simulink model "sim_discrete_planar_7dof"  (R2023b)
settings: Solver=VariableStepAuto  StartTime=0.0  StopTime=T_sim  FixedStep=param_global.Ta  RelTol=1e-3
InitFcn:
  | parameters_7dof;
undefined symbols (not defined in the file): fx, fy, fz, init_bus_param, param_global, param_robot, param_vis, path_param, q_0, q_0_p, tau_x, tau_y, tau_z
(part 1 of 2)
settings Model: Creator=emu  LastModifiedBy=emu
settings DebuggingCC: ReadBeforeWriteMsg=DisableAll  WriteAfterWriteMsg=DisableAll  WriteAfterReadMsg=DisableAll  MultiTaskDSMMsg=none
settings ModelReferenceCC: UpdateModelReferenceTargets=IfOutOfDate
settings SFSimCC: SFSimEcho=off

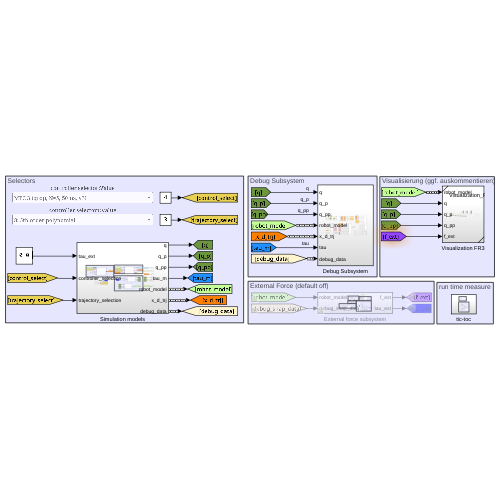
[thumbnail: Simulink's stored preview of the top-level diagram]
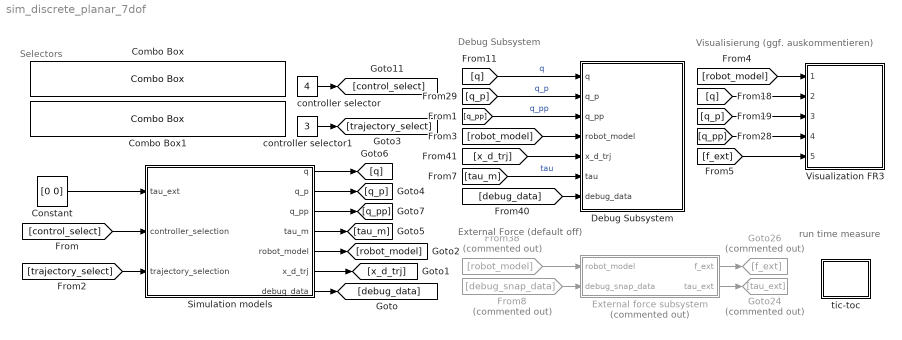
== system sim_discrete_planar_7dof ==
  note: run time measure
  note: Selectors
  note: Visualisierung (ggf. auskommentieren)
  note: Debug Subsystem
  note: External Force (default off)
  Combo Box : ComboBox  SelectedLabel=MPC 3 (qrqp, N=5, 50ms, v3)
      settings: Values={{'Cartesian CT Control', 'MPC 1 (ipopt, N=5, 20ms, v2)', 'MPC 2 (qrqp, N=5, 20ms, v2)', 'MPC 3 (qrqp, N=5, 50ms, v3)', 'MPC 4 (qrqp, N=5, 1ms, v1)', 'MPC 5 (qrqp, N=5, 10ms, v4'}, [1 2 3 4 5 6]}
  Combo Box1 : ComboBox  SelectedLabel=3: 5th order polynomial
      settings: Values={{'1: stabilize equilibrium', '2: 5th order differential filter', '3: 5th order polynomial', '4: smooth sinus'}, [1 2 3 4]}
  Constant : Constant  Value=[0 0]
  Debug Subsystem : Subsystem
  External force subsystem : Subsystem  Commented=on
  From38 : From  Commented=on  GotoTag=robot_model
  From8 : From  Commented=on  GotoTag=debug_snap_data
  Goto24 : Goto  Commented=on  GotoTag=tau_ext
  Goto26 : Goto  Commented=on  GotoTag=f_ext
  Simulation models : Subsystem
  Visualization FR3 : Subsystem  ReferencedSubsystem=Visualization_FR3_shared_subsystem
  controller selector : Constant  Value=4  OutDataTypeStr=uint32  SampleTime=-1
  controller selector1 : Constant  Value=3  OutDataTypeStr=uint32  SampleTime=-1
  tic-toc : Subsystem
  wires:
  controller selector/1 -> [control_select]
  [tau_m] -> Debug Subsystem/6(tau)  "tau"
  [debug_data] -> Debug Subsystem/7(debug_data)
  External force subsystem/1(f_ext) -> Goto26/1
  [q_p] -> Debug Subsystem/2(q_p)  "q_p"
  [robot_model] -> Debug Subsystem/4(robot_model)
  [robot_model] -> Visualization FR3/1
  From8/1 -> External force subsystem/2(debug_snap_data)
  [q_pp] -> Visualization FR3/4
  [f_ext] -> Visualization FR3/5
  [x_d_trj] -> Debug Subsystem/5(x_d_trj)
  From38/1 -> External force subsystem/1(robot_model)
  [q_p] -> Visualization FR3/3
  External force subsystem/2(tau_ext) -> Goto24/1
  [q] -> Visualization FR3/2
  [q] -> Debug Subsystem/1(q)  "q"
  [q_pp] -> Debug Subsystem/3(q_pp)  "q_pp"
  Simulation models/7(debug_data) -> [debug_data]
  Simulation models/6(x_d_trj) -> [x_d_trj]
  Simulation models/5(robot_model) -> [robot_model]
  Simulation models/4(tau_m) -> [tau_m]
  Simulation models/3(q_pp) -> [q_pp]
  Simulation models/2(q_p) -> [q_p]
  Simulation models/1(q) -> [q]
  [control_select] -> Simulation models/2(controller_selection)
  Constant/1 -> Simulation models/1(tau_ext)
  controller selector1/1 -> [trajectory_select]
  [trajectory_select] -> Simulation models/3(trajectory_selection)

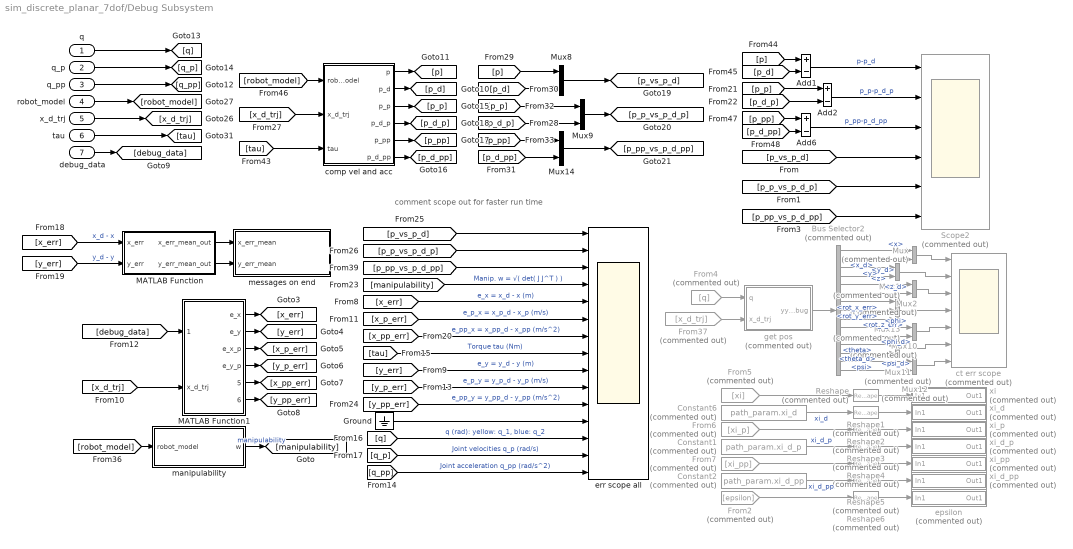
== system sim_discrete_planar_7dof/Debug Subsystem ==
  note: comment scope out for faster run time
  q : Inport
  q_p : Inport  Port=2
  q_pp : Inport  Port=3
  robot_model : Inport  Port=4
  x_d_trj : Inport  Port=5
  tau : Inport  Port=6
  debug_data : Inport  Port=7  OutDataTypeStr=Bus: debug_data_bus
  Add1 : Sum  Inputs=+-
  Add2 : Sum  Inputs=+-
  Add6 : Sum  Inputs=+-
  Bus Selector2 : BusSelector  Commented=on  OutputSignals=x,x_d,y,y_d,z,z_d,rot_x_err,rot_y_err,rot_z_err,phi,phi_d,theta,theta_d,psi,psi_d
  Constant1 : Constant  Commented=on  Value=path_param.xi_d_p  SampleTime=-1
  Constant2 : Constant  Commented=on  Value=path_param.xi_d_pp  SampleTime=-1
  Constant6 : Constant  Commented=on  Value=path_param.xi_d  SampleTime=-1
  From2 : From  Commented=on  GotoTag=epsilon
  From37 : From  Commented=on  GotoTag=x_d_trj
  From4 : From  Commented=on  GotoTag=q
  From5 : From  Commented=on  GotoTag=xi
  From6 : From  Commented=on  GotoTag=xi_p
  From7 : From  Commented=on  GotoTag=xi_pp
  Ground : Ground
  MATLAB Function : MATLAB Function  TreatAsAtomicUnit=on
  MATLAB Function1 : MATLAB Function  TreatAsAtomicUnit=on
  Mux{,1..2,10..12} (6 alike) : Mux  Commented=on  Inputs=2
  Mux13 : Mux  Commented=on  Inputs=3
  Mux14 : Mux  Inputs=2
  Mux8 : Mux  Inputs=2
  Mux9 : Mux  Inputs=2
  Reshape{,1..6} (7 alike) : Reshape  Commented=on
  Scope2 : Scope  Commented=on  NumInputPorts=6
  comp vel and acc : MATLAB Function  TreatAsAtomicUnit=on
  ct err scope : Scope  Commented=on  NumInputPorts=7
  epsilon : Subsystem  Commented=on
  err scope all : Scope  NumInputPorts=15
  get pos : MATLAB Function  Commented=on  TreatAsAtomicUnit=on  SystemSampleTime=param_global.Ta
  manipulability : MATLAB Function  TreatAsAtomicUnit=on
  messages on end : Subsystem
  xi : Subsystem  Commented=on
  xi_d : Subsystem  Commented=on
  xi_d_p : Subsystem  Commented=on
  xi_d_pp : Subsystem  Commented=on
  xi_p : Subsystem  Commented=on
  xi_pp : Subsystem  Commented=on
  wires:
  [robot_model] -> manipulability/1(robot_model)
  q/1 -> [q]
  q_p/1 -> [q_p]
  q_pp/1 -> [q_pp]
  From4/1 -> get pos/1(q)
  Constant6/1 -> Reshape1/1  "xi_d"
  Constant1/1 -> Reshape3/1  "xi_d_p"
  Constant2/1 -> Reshape5/1  "xi_d_pp"
  From5/1 -> Reshape/1
  From6/1 -> Reshape2/1
  From7/1 -> Reshape4/1
  x_d_trj/1 -> [x_d_trj]
  robot_model/1 -> [robot_model]
  debug_data/1 -> [debug_data]
  tau/1 -> [tau]
  From37/1 -> get pos/2(x_d_trj)
  get pos/1(yy_debug) -> Bus Selector2/1
  Mux/1 -> ct err scope/1
  Mux1/1 -> ct err scope/2
  Mux2/1 -> ct err scope/3
  Mux10/1 -> ct err scope/5
  Mux11/1 -> ct err scope/6
  Mux12/1 -> ct err scope/7
  Mux13/1 -> ct err scope/4
  Bus Selector2/1 -> Mux/1  "<x>"
  Bus Selector2/2 -> Mux/2  "<x_d>"
  Bus Selector2/3 -> Mux1/1  "<y>"
  Bus Selector2/4 -> Mux1/2  "<y_d>"
  Bus Selector2/5 -> Mux2/1  "<z>"
  Bus Selector2/6 -> Mux2/2  "<z_d>"
  Bus Selector2/7 -> Mux13/1  "<rot_x_err>"
  Bus Selector2/8 -> Mux13/2  "<rot_y_err>"
  Bus Selector2/9 -> Mux13/3  "<rot_z_err>"
  Bus Selector2/10 -> Mux10/1  "<phi>"
  Bus Selector2/11 -> Mux10/2  "<phi_d>"
  Bus Selector2/12 -> Mux11/1  "<theta>"
  Bus Selector2/13 -> Mux11/2  "<theta_d>"
  Bus Selector2/14 -> Mux12/1  "<psi>"
  Bus Selector2/15 -> Mux12/2  "<psi_d>"
  Reshape/1 -> xi/1(In1)
  Reshape1/1 -> xi_d/1(In1)
  Reshape2/1 -> xi_p/1(In1)
  Reshape3/1 -> xi_d_p/1(In1)
  Reshape4/1 -> xi_pp/1(In1)
  Reshape5/1 -> xi_d_pp/1(In1)
  From2/1 -> Reshape6/1
  Reshape6/1 -> epsilon/1(In1)
  manipulability/1(w) -> [manipulability]  "manipulability"
  [x_err] -> MATLAB Function/1(x_err)  "x_d - x"
  [y_err] -> MATLAB Function/2(y_err)  "y_d - y"
  MATLAB Function/2(y_err_mean_out) -> messages on end/2(y_err_mean)
  MATLAB Function/1(x_err_mean_out) -> messages on end/1(x_err_mean)
  [debug_data] -> MATLAB Function1/1(debug_data)
  [x_d_trj] -> MATLAB Function1/2(x_d_trj)
  MATLAB Function1/1(e_x) -> [x_err]
  MATLAB Function1/2(e_y) -> [y_err]
  MATLAB Function1/3(e_x_p) -> [x_p_err]
  MATLAB Function1/4(e_y_p) -> [y_p_err]
  MATLAB Function1/5(e_x_pp) -> [x_pp_err]
  MATLAB Function1/6(e_y_pp) -> [y_pp_err]
  [manipulability] -> err scope all/4  "Manip. w = √( det( J J^T ) )"
  [tau] -> err scope all/8  "Torque tau (Nm)"
  [x_err] -> err scope all/5  "e_x = x_d - x (m)"
  [y_err] -> err scope all/9  "e_y = y_d - y (m)"
  [x_p_err] -> err scope all/6  "e_p_x = x_p_d - x_p (m/s)"
  [y_p_err] -> err scope all/10  "e_p_y = y_p_d - y_p (m/s)"
  [x_pp_err] -> err scope all/7  "e_pp_x = x_pp_d - x_pp (m/s^2)"
  [y_pp_err] -> err scope all/11  "e_pp_y = y_pp_d - y_pp (m/s^2)"
  [q] -> err scope all/13  "q (rad): yellow: q_1, blue: q_2"
  [q_p] -> err scope all/14  "Joint velocities q_p (rad/s)"
  [q_pp] -> err scope all/15  "Joint acceleration q_pp (rad/s^2)"
  [p_d_p] -> Mux9/2
  [tau] -> comp vel and acc/3(tau)
  [p_p] -> Mux9/1
  [p_d] -> Mux8/2
  [x_d_trj] -> comp vel and acc/2(x_d_trj)
  [p] -> Mux8/1
  [p_pp] -> Mux14/1
  [p_d_pp] -> Mux14/2
  [robot_model] -> comp vel and acc/1(robot_model)
  comp vel and acc/2(p_d) -> [p_d]
  comp vel and acc/1(p) -> [p]
  comp vel and acc/3(p_p) -> [p_p]
  comp vel and acc/6(p_d_pp) -> [p_d_pp]
  comp vel and acc/5(p_pp) -> [p_pp]
  comp vel and acc/4(p_d_p) -> [p_d_p]
  [p_pp] -> Add6/1
  [p] -> Add1/1
  [p_d] -> Add1/2
  [p_d_p] -> Add2/2
  [p_p] -> Add2/1
  Add6/1 -> Scope2/3  "p_pp-p_d_pp"
  Add2/1 -> Scope2/2  "p_p-p_d_p"
  Add1/1 -> Scope2/1  "p-p_d"
  [p_d_pp] -> Add6/2
  [p_p_vs_p_d_p] -> err scope all/2
  [p_vs_p_d] -> err scope all/1
  [p_pp_vs_p_d_pp] -> err scope all/3
  Ground/1 -> err scope all/12
  Mux8/1 -> [p_vs_p_d]
  Mux9/1 -> [p_p_vs_p_d_p]
  Mux14/1 -> [p_pp_vs_p_d_pp]
  [p_vs_p_d] -> Scope2/4
  [p_p_vs_p_d_p] -> Scope2/5
  [p_pp_vs_p_d_pp] -> Scope2/6

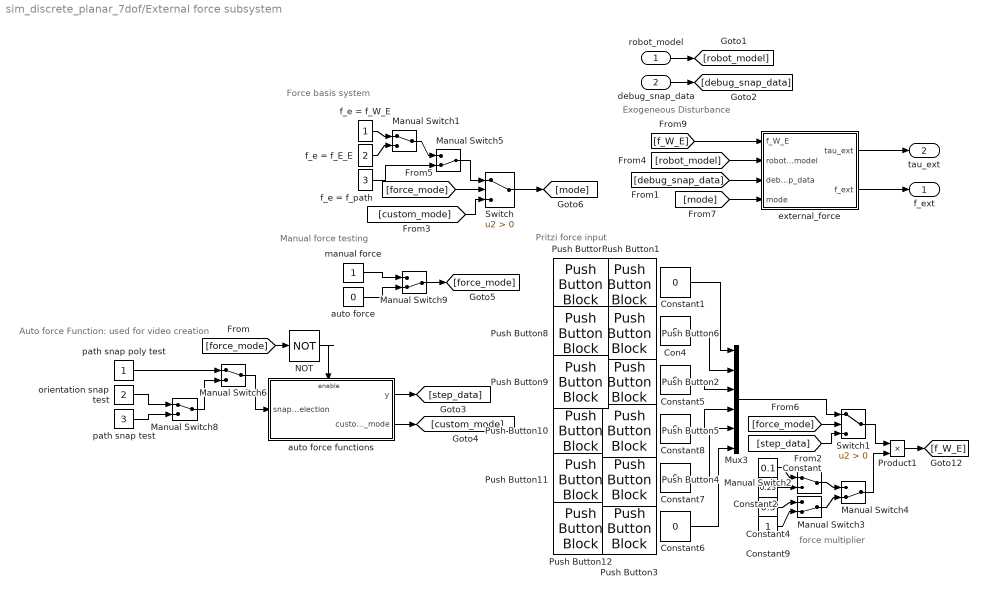
== system sim_discrete_planar_7dof/External force subsystem ==
  note: Force basis system
  note: Manual force testing
  note: Auto force Function: used for video creation
  note: force multiplier
  note: Exogeneous Disturbance
  note: Pritzi force input
  robot_model : Inport
  debug_snap_data : Inport  Port=2  OutDataTypeStr=Bus: debug_snap_data_bus
  Con4 : Constant  Value=0  SampleTime=-1
  Constant : Constant  Value=0.1  SampleTime=-1
  Constant{1,5..8} (5 alike) : Constant  Value=0  SampleTime=-1
  Constant2 : Constant  Value=0.25  SampleTime=-1
  Constant4 : Constant  Value=0.5  SampleTime=-1
  Constant9 : Constant  SampleTime=-1
  Manual Switch{1..2,6,8} (4 alike) : ManualSwitch
  Manual Switch{3..5,9} (4 alike) : ManualSwitch  CurrentSetting=0
  Mux3 : Mux  Inputs=6
  NOT : Logic  Operator=NOT  IconShape=distinctive  AllPortsSameDT=off  OutDataTypeStr=boolean
  Product1 : Product
  Push Button1 : PushButtonBlock  ButtonText=fx  OnValue=20  OffValue=0.000000
  Push Button10 : PushButtonBlock  ButtonText=-tau_x  OnValue=-1  OffValue=0.000000
  Push Button11 : PushButtonBlock  ButtonText=-tau_y  OnValue=-1  OffValue=0.000000
  Push Button12 : PushButtonBlock  ButtonText=-tau_z  OnValue=-1  OffValue=0.000000
  Push Button2 : PushButtonBlock  ButtonText=fz  OnValue=20  OffValue=0.000000
  Push Button3 : PushButtonBlock  ButtonText=tau_z  OffValue=0.000000
  Push Button4 : PushButtonBlock  ButtonText=tau_y  OffValue=0.000000
  Push Button5 : PushButtonBlock  ButtonText=tau_x  OffValue=0.000000
  Push Button6 : PushButtonBlock  ButtonText=fy  OnValue=20  OffValue=0.000000
  Push Button7 : PushButtonBlock  ButtonText=-fx  OnValue=-20  OffValue=0.000000
  Push Button8 : PushButtonBlock  ButtonText=-fy  OnValue=-20  OffValue=0.000000
  Push Button9 : PushButtonBlock  ButtonText=-fz  OnValue=-20  OffValue=0.000000
  Switch : Switch  Criteria=u2 > Threshold  SaturateOnIntegerOverflow=off  InputSameDT=off
  Switch1 : Switch  Criteria=u2 > Threshold  SaturateOnIntegerOverflow=off  InputSameDT=off
  auto force : Constant  Value=0
  auto force functions : Subsystem
  external_force : MATLAB Function  TreatAsAtomicUnit=on
  f_e = f_E_E : Constant  Value=2  SampleTime=-1
  f_e = f_W_E : Constant  SampleTime=-1
  f_e = f_path : Constant  Value=3  SampleTime=-1
  manual force : Constant
  orientation snap test : Constant  Value=2
  path snap poly test : Constant
  path snap test : Constant  Value=3
  f_ext : Outport
  tau_ext : Outport  Port=2
  wires:
  Product1/1 -> [f_W_E]
  Constant4/1 -> Manual Switch3/1
  Constant6/1 -> Mux3/6
  Constant5/1 -> Mux3/3
  Constant/1 -> Manual Switch2/1
  Constant8/1 -> Mux3/4
  [f_W_E] -> external_force/1(f_W_E)
  external_force/2(f_ext) -> f_ext/1
  Constant9/1 -> Manual Switch3/2
  Manual Switch2/1 -> Manual Switch4/1
  Con4/1 -> Mux3/2
  [robot_model] -> external_force/2(robot_model)
  Manual Switch4/1 -> Product1/2
  Constant1/1 -> Mux3/1
  f_e = f_W_E/1 -> Manual Switch1/1
  Constant7/1 -> Mux3/5
  Constant2/1 -> Manual Switch2/2
  f_e = f_E_E/1 -> Manual Switch1/2
  Manual Switch3/1 -> Manual Switch4/2
  external_force/1(tau_ext) -> tau_ext/1
  Manual Switch1/1 -> Manual Switch5/1
  f_e = f_path/1 -> Manual Switch5/2
  robot_model/1 -> [robot_model]
  debug_snap_data/1 -> [debug_snap_data]
  [debug_snap_data] -> external_force/3(debug_snap_data)
  Switch1/1 -> Product1/1
  Manual Switch5/1 -> Switch/1
  [custom_mode] -> Switch/3
  auto force functions/1(y) -> [step_data]
  auto force functions/2(custom_mode) -> [custom_mode]
  Manual Switch6/1 -> auto force functions/1(snap selection)
  path snap test/1 -> Manual Switch8/2
  orientation snap test/1 -> Manual Switch8/1
  manual force/1 -> Manual Switch9/1
  auto force/1 -> Manual Switch9/2
  Manual Switch9/1 -> [force_mode]
  [force_mode] -> Switch/2
  [force_mode] -> Switch1/2
  [step_data] -> Switch1/3
  Mux3/1 -> Switch1/1
  Switch/1 -> [mode]
  [mode] -> external_force/4(mode)
  Manual Switch8/1 -> Manual Switch6/2
  path snap poly test/1 -> Manual Switch6/1
  [force_mode] -> NOT/1
  NOT/1 -> auto force functions/Enable

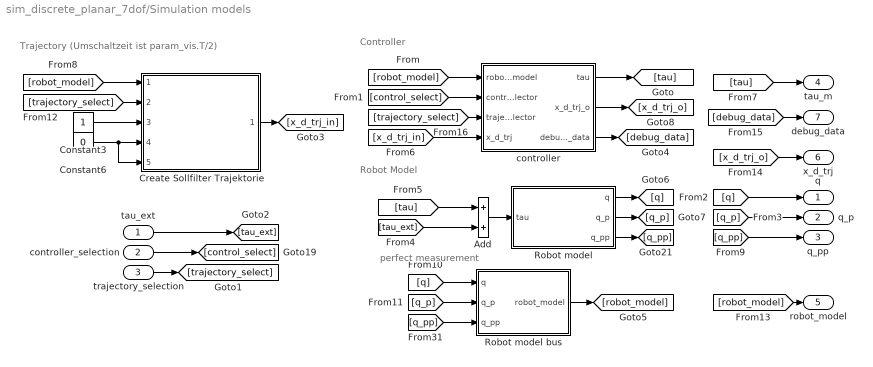
== system sim_discrete_planar_7dof/Simulation models ==
  note: Controller
  note: Trajectory (Umschaltzeit ist param_vis.T/2)
  note: Robot Model
  note: perfect measurement
  tau_ext : Inport
  controller_selection : Inport  Port=2
  trajectory_selection : Inport  Port=3
  Add : Sum
  Constant3 : Constant
  Constant6 : Constant  Value=0
  Create Sollfilter Trajektorie : Subsystem  ReferencedSubsystem=trajectory_generation_ref_subsys
  Robot model : Subsystem
  Robot model bus : MATLAB Function  TreatAsAtomicUnit=on
  controller : Subsystem
  q : Outport
  q_p : Outport  Port=2
  q_pp : Outport  Port=3
  tau_m : Outport  Port=4
  robot_model : Outport  Port=5  OutDataTypeStr=Bus: robot_model
  x_d_trj : Outport  Port=6  OutDataTypeStr=Bus: x_d
  debug_data : Outport  Port=7  OutDataTypeStr=Bus: debug_data_bus
  wires:
  [q_p] -> Robot model bus/2(q_p)
  Robot model/2(q_p) -> [q_p]
  [tau_ext] -> Add/2
  Robot model/3(q_pp) -> [q_pp]
  [q] -> Robot model bus/1(q)
  [q_pp] -> Robot model bus/3(q_pp)
  Robot model/1(q) -> [q]
  [robot_model] -> Create Sollfilter Trajektorie/1
  [tau] -> Add/1
  Robot model bus/1(robot_model) -> [robot_model]
  tau_ext/1 -> [tau_ext]
  controller_selection/1 -> [control_select]
  [q_pp] -> q_pp/1
  [q_p] -> q_p/1
  [x_d_trj_o] -> x_d_trj/1
  [debug_data] -> debug_data/1
  [q] -> q/1
  [robot_model] -> robot_model/1
  [tau] -> tau_m/1
  controller/3(debug_data) -> [debug_data]
  [robot_model] -> controller/1(robot_model)
  [control_select] -> controller/2(controller_selector)
  [x_d_trj_in] -> controller/4(x_d_trj)
  controller/1(tau) -> [tau]
  Constant3/1 -> Create Sollfilter Trajektorie/3
  Constant6/1 -> Create Sollfilter Trajektorie/5, Create Sollfilter Trajektorie/4
  Create Sollfilter Trajektorie/1 -> [x_d_trj_in]
  trajectory_selection/1 -> [trajectory_select]
  [trajectory_select] -> Create Sollfilter Trajektorie/2
  controller/2(x_d_trj_o) -> [x_d_trj_o]
  [trajectory_select] -> controller/3(trajectory selector)
  Add/1 -> Robot model/1(tau)

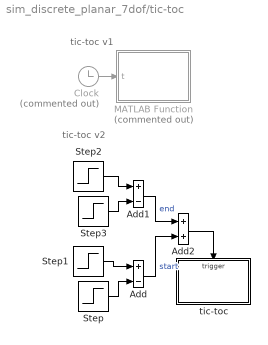
== system sim_discrete_planar_7dof/tic-toc ==
  note: tic-toc v1
  note: tic-toc v2
  Add : Sum  Inputs=+-
  Add1 : Sum  Inputs=+-
  Add2 : Sum
  Clock : Clock  Commented=on
  MATLAB Function : MATLAB Function  Commented=on  TreatAsAtomicUnit=on
  Step : Step  Time=param_global.Ta*2  SampleTime=param_global.Ta
  Step1 : Step  Time=param_global.Ta  SampleTime=param_global.Ta
  Step2 : Step  Time=param_vis.T-param_global.Ta  SampleTime=param_global.Ta
  Step3 : Step  Time=param_vis.T  SampleTime=param_global.Ta
  tic-toc : Subsystem  TreatAsAtomicUnit=on
  wires:
  Add/1 -> Add2/2  "start"
  Step2/1 -> Add1/1
  Add2/1 -> tic-toc/Trigger
  Step3/1 -> Add1/2
  Add1/1 -> Add2/1  "end"
  Step1/1 -> Add/1
  Step/1 -> Add/2
  Clock/1 -> MATLAB Function/1(t)

== system sim_discrete_planar_7dof/Debug Subsystem/epsilon ==
  In1 : Inport
  Out1 : Outport
  wires:
  In1/1 -> Out1/1

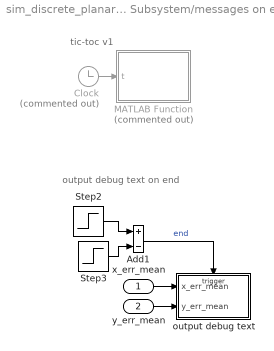
== system sim_discrete_planar_7dof/Debug Subsystem/messages on end ==
  note: tic-toc v1
  note: output debug text on end
  x_err_mean : Inport
  y_err_mean : Inport  Port=2
  Add1 : Sum  Inputs=+-
  Clock : Clock  Commented=on
  MATLAB Function : MATLAB Function  Commented=on  TreatAsAtomicUnit=on
  Step2 : Step  Time=param_vis.T-param_global.Ta  SampleTime=param_global.Ta
  Step3 : Step  Time=param_vis.T  SampleTime=param_global.Ta
  output debug text : Subsystem  TreatAsAtomicUnit=on
  wires:
  Clock/1 -> MATLAB Function/1(t)
  Add1/1 -> output debug text/Trigger  "end"
  Step3/1 -> Add1/2
  Step2/1 -> Add1/1
  y_err_mean/1 -> output debug text/2(y_err_mean)
  x_err_mean/1 -> output debug text/1(x_err_mean)

== system sim_discrete_planar_7dof/Debug Subsystem/xi ==
  In1 : Inport
  Out1 : Outport
  wires:
  In1/1 -> Out1/1

== system sim_discrete_planar_7dof/Debug Subsystem/xi_d ==
  In1 : Inport
  Out1 : Outport
  wires:
  In1/1 -> Out1/1

== system sim_discrete_planar_7dof/Debug Subsystem/xi_d_p ==
  In1 : Inport
  Out1 : Outport
  wires:
  In1/1 -> Out1/1

== system sim_discrete_planar_7dof/Debug Subsystem/xi_d_pp ==
  In1 : Inport
  Out1 : Outport
  wires:
  In1/1 -> Out1/1

== system sim_discrete_planar_7dof/Debug Subsystem/xi_p ==
  In1 : Inport
  Out1 : Outport
  wires:
  In1/1 -> Out1/1

== system sim_discrete_planar_7dof/Debug Subsystem/xi_pp ==
  In1 : Inport
  Out1 : Outport
  wires:
  In1/1 -> Out1/1

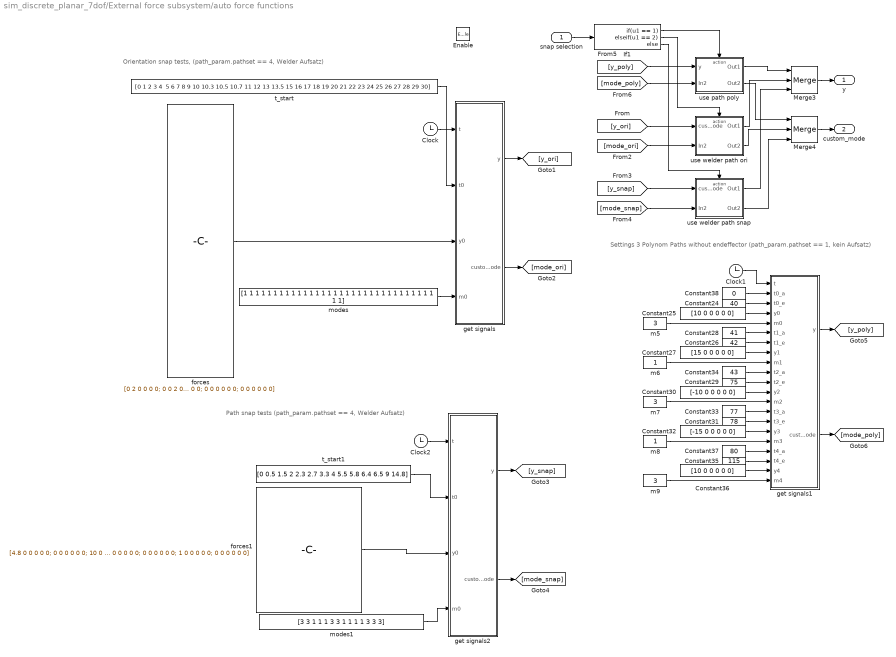
== system sim_discrete_planar_7dof/External force subsystem/auto force functions ==
  note: Orientation snap tests, (path_param.pathset == 4, Welder Aufsatz)
  note: Path snap tests (path_param.pathset == 4, Welder Aufsatz)
  note: Settings 3 Polynom Paths without endeffector
      | (path_param.pathset == 1, kein Aufsatz)
  snap selection : Inport
  Enable : EnablePort
  Clock : Clock
  Clock1 : Clock
  Clock2 : Clock
  Constant24 : Constant  Value=40
  Constant25 : Constant  Value=[10 0 0 0 0 0]
  Constant26 : Constant  Value=42
  Constant27 : Constant  Value=[15 0 0 0 0 0]
  Constant28 : Constant  Value=41
  Constant29 : Constant  Value=75
  Constant30 : Constant  Value=[-10 0 0 0 0 0]
  Constant31 : Constant  Value=78
  Constant32 : Constant  Value=[-15 0 0 0 0 0]
  Constant33 : Constant  Value=77
  Constant34 : Constant  Value=43
  Constant35 : Constant  Value=115
  Constant36 : Constant  Value=[10 0 0 0 0 0]
  Constant37 : Constant  Value=80
  Constant38 : Constant  Value=0
  If1 : If  IfExpression=u1 == 1  ElseIfExpressions=u1 == 2
  Merge3 : Merge  Inputs=3
  Merge4 : Merge  Inputs=3
  forces : Constant  Value=|
      | [0 2 0 0 0 0;
      | 0 0 2 0 0 0;
      | 0 -2 0 0 0 0;
      | 0 0 -2 0 0 0;
      | 30 0 7 0 0 0;
      | 0 2 0 0 0 0;
      | 0 0 2 0 0 0;
      | 0 -2 0 0 0 0;
      | 0 0 -2 0 0 0;
      | 0 0 0 0 0 0;
      | 0 0 0 0.25 0 0;
      | 0 0 0 0.26 0 0;
      | 0 0 0 0.27 0 0;
      | 0 0 0 0 0 0;
      | 0 -2 0 0 0 0;
      | 0 0 0 0 0 0;
      | 0 0 0 0.26 0 0;
      | 0 0 0 0 0 0;
      | 0 -2 0 0 0 0;
      | 0 0 2 0 0 0;
      | 0 2 0 0 0 0;
      | 0 0 -2 0 0 0;
      | -30 3.5 -3.5 0 0 0;
      | 0 -2 0 0 0 0;
      | 0 0 2 0 0 0;
      | 0 2 0 0 0 0;
      | 0 0 -2 0 0 0;
      | 0 0 0 0 0 0;
      | 0 0 0 0 0 0;
      | 0 0 0 0 0 0;
      | 0 0 0 0 0 0;
      | 0 0 0 0 0 0;
      | 0 0 0 0 0 0;
      | 0 0 0 0 0 0]
  forces1 : Constant  Value=|
      | [4.8 0 0 0 0 0;
      | 0 0 0 0 0 0;
      | 10 0 0 0 0 0;
      | 15 0 3 0 0 0
      | 10 0 3 0 0 0;
      | 0 0 0 0 0 0;
      | 1 0 0 0 0 0;
      | 0 0 0 0 0 0;
      | 15 0 0 0 0 0;
      | 10 -3 0 0 0 0
      | 10 0 0 0 0 0;
      | 0 0 0 0 0 0;
      | 1 0 0 0 0 0;
      | 0 0 0 0 0 0]
  get signals : MATLAB Function  TreatAsAtomicUnit=on
  get signals1 : MATLAB Function  TreatAsAtomicUnit=on
  get signals2 : MATLAB Function  TreatAsAtomicUnit=on
  m5 : Constant  Value=3
  m6 : Constant
  m7 : Constant  Value=3
  m8 : Constant
  m9 : Constant  Value=3
  modes : Constant  Value=[1 1 1 1 1 1 1 1 1 1 1 1 1 1 1 1 1 1 1 1 1 1 1 1 1 1 1 1 1 1 1 1 1 1]
  modes1 : Constant  Value=[3 3 1 1 1 3 3 1 1 1 1 3 3 3]
  t_start : Constant  Value="[0 1 2 3 4  5 6 7 8 9 10 10.3 10.5 10.7 11 12 13 13.5 15 16 17 18 19 20 21 22 23 24 25 26 27 28 29 30]"
  t_start1 : Constant  Value="[0 0.5 1.5 2 2.3  2.7 3.3 4 5.5  5.8 6.4 6.5 9 14.8]"
  use path poly : Subsystem  TreatAsAtomicUnit=on
  use welder path ori : Subsystem  TreatAsAtomicUnit=on
  use welder path snap : Subsystem  TreatAsAtomicUnit=on
  y : Outport
  custom_mode : Outport  Port=2
  wires:
  Constant26/1 -> get signals1/7(t1_e)
  Constant36/1 -> get signals1/20(y4)
  Constant34/1 -> get signals1/10(t2_a)
  Constant29/1 -> get signals1/11(t2_e)
  Constant37/1 -> get signals1/18(t4_a)
  Constant33/1 -> get signals1/14(t3_a)
  Constant35/1 -> get signals1/19(t4_e)
  Clock/1 -> get signals/1(t)
  m5/1 -> get signals1/5(m0)
  m8/1 -> get signals1/17(m3)
  m7/1 -> get signals1/13(m2)
  m9/1 -> get signals1/21(m4)
  Constant32/1 -> get signals1/16(y3)
  Clock1/1 -> get signals1/1(t)
  m6/1 -> get signals1/9(m1)
  Constant25/1 -> get signals1/4(y0)
  Constant38/1 -> get signals1/2(t0_a)
  Constant31/1 -> get signals1/15(t3_e)
  Constant28/1 -> get signals1/6(t1_a)
  Constant27/1 -> get signals1/8(y1)
  Constant24/1 -> get signals1/3(t0_e)
  Constant30/1 -> get signals1/12(y2)
  use path poly/1(Out1) -> Merge3/1
  use welder path ori/1(Out1) -> Merge3/2
  use path poly/2(Out2) -> Merge4/1
  use welder path ori/2(Out2) -> Merge4/2
  Merge4/1 -> custom_mode/1
  Merge3/1 -> y/1
  If1/1 -> use path poly/Action
  t_start/1 -> get signals/2(t0)
  forces/1 -> get signals/3(y0)
  modes/1 -> get signals/4(m0)
  t_start1/1 -> get signals2/2(t0)
  forces1/1 -> get signals2/3(y0)
  modes1/1 -> get signals2/4(m0)
  Clock2/1 -> get signals2/1(t)
  snap selection/1 -> If1/1
  If1/2 -> use welder path ori/Action
  If1/3 -> use welder path snap/Action
  use welder path snap/1(Out1) -> Merge3/3
  use welder path snap/2(Out2) -> Merge4/3
  get signals1/1(y) -> [y_poly]
  get signals1/2(custom_mode) -> [mode_poly]
  get signals2/1(y) -> [y_snap]
  get signals2/2(custom_mode) -> [mode_snap]
  get signals/1(y) -> [y_ori]
  get signals/2(custom_mode) -> [mode_ori]
  [y_poly] -> use path poly/1(y)
  [mode_poly] -> use path poly/2(In2)
  [y_ori] -> use welder path ori/1(custom_mode)
  [mode_ori] -> use welder path ori/2(In2)
  [y_snap] -> use welder path snap/1(custom_mode)
  [mode_snap] -> use welder path snap/2(In2)

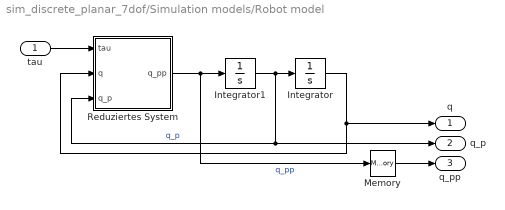
== system sim_discrete_planar_7dof/Simulation models/Robot model ==
  tau : Inport
  Integrator : Integrator  InitialCondition=q_0
  Integrator1 : Integrator  InitialCondition=q_0_p
  Memory : Memory  InitialCondition=zeros(2,1)  InheritSampleTime=on
  Reduziertes System : MATLAB Function
  q : Outport
  q_p : Outport  Port=2
  q_pp : Outport  Port=3
  wires:
  Integrator/1 -> q/1, Reduziertes System/2(q)
  Integrator1/1 -> q_p/1, Reduziertes System/3(q_p), Integrator/1  "q_p"
  Reduziertes System/1(q_pp) -> Memory/1, Integrator1/1  "q_pp"
  tau/1 -> Reduziertes System/1(tau)
  Memory/1 -> q_pp/1

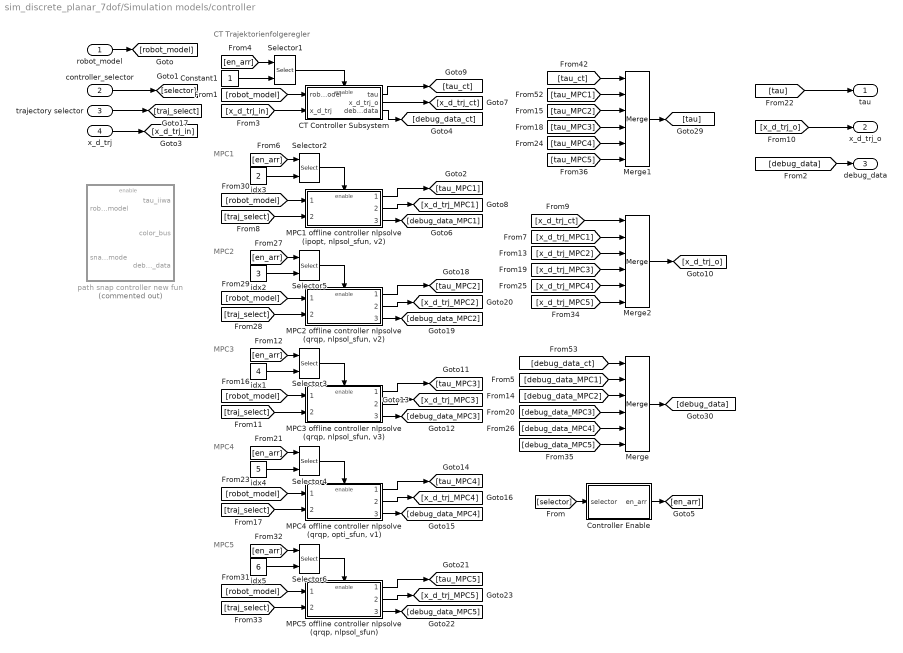
== system sim_discrete_planar_7dof/Simulation models/controller ==
  note: CT Trajektorienfolgeregler
  note: MPC1
  note: MPC2
  note: MPC3
  note: MPC4
  note: MPC5
  robot_model : Inport  OutDataTypeStr=Bus: robot_model
  controller_selector : Inport  Port=2
  trajectory selector : Inport  Port=3
  x_d_trj : Inport  Port=4  OutDataTypeStr=Bus: x_d
  CT Controller Subsystem : Subsystem
  Constant1 : Constant
  Controller Enable : MATLAB Function  TreatAsAtomicUnit=on
  "MPC1 offline controller nlpsolve (ipopt, nlpsol_sfun, v2)" : Subsystem  ReferencedSubsystem=MPC1_nlpsol
  "MPC2 offline controller nlpsolve (qrqp, nlpsol_sfun, v2)" : Subsystem  ReferencedSubsystem=MPC2_opti
  "MPC3 offline controller nlpsolve (qrqp, nlpsol_sfun, v3)" : Subsystem  ReferencedSubsystem=MPC3_opti
  "MPC4 offline controller nlpsolve (qrqp, opti_sfun, v1)" : Subsystem  ReferencedSubsystem=MPC4_opti
  "MPC5 offline controller nlpsolve (qrqp, nlpsol_sfun)" : Subsystem  ReferencedSubsystem=MPC5_nlpsol
  Merge : Merge  Inputs=6
  Merge1 : Merge  Inputs=6
  Merge2 : Merge  Inputs=6
  Selector{1..6} (6 alike) : Selector  IndexOptions=Index vector (port)  Indices=[1 3]  OutputSizes=1
  idx1 : Constant  Value=4
  idx2 : Constant  Value=3
  idx3 : Constant  Value=2
  idx4 : Constant  Value=5
  idx5 : Constant  Value=6
  path snap controller new fun : Subsystem  Commented=on
  tau : Outport
  x_d_trj_o : Outport  Port=2  OutDataTypeStr=Bus: x_d
  debug_data : Outport  Port=3  OutDataTypeStr=Bus: debug_data_bus
  wires:
  [robot_model] -> CT Controller Subsystem/1(robot_model)
  [debug_data] -> debug_data/1
  controller_selector/1 -> [selector]
  [tau] -> tau/1
  x_d_trj/1 -> [x_d_trj_in]
  [x_d_trj_in] -> CT Controller Subsystem/2(x_d_trj)
  Controller Enable/1(en_arr) -> [en_arr]
  [selector] -> Controller Enable/1(selector)
  robot_model/1 -> [robot_model]
  [debug_data_ct] -> Merge/1
  [tau_ct] -> Merge1/1
  [tau_MPC1] -> Merge1/2
  Merge1/1 -> [tau]
  Merge/1 -> [debug_data]
  [debug_data_MPC1] -> Merge/2
  CT Controller Subsystem/1(tau) -> [tau_ct]
  Selector1/1 -> CT Controller Subsystem/Enable
  Constant1/1 -> Selector1/2
  [en_arr] -> Selector1/1
  CT Controller Subsystem/3(debug_data) -> [debug_data_ct]
  CT Controller Subsystem/2(x_d_trj_o) -> [x_d_trj_ct]
  [x_d_trj_ct] -> Merge2/1
  [x_d_trj_MPC1] -> Merge2/2
  Merge2/1 -> [x_d_trj_o]
  [x_d_trj_o] -> x_d_trj_o/1
  [tau_MPC2] -> Merge1/3
  [debug_data_MPC2] -> Merge/3
  [x_d_trj_MPC2] -> Merge2/3
  [debug_data_MPC3] -> Merge/4
  [x_d_trj_MPC3] -> Merge2/4
  [tau_MPC3] -> Merge1/4
  [tau_MPC4] -> Merge1/5
  [x_d_trj_MPC4] -> Merge2/5
  [debug_data_MPC4] -> Merge/5
  trajectory selector/1 -> [traj_select]
  [traj_select] -> "MPC1 offline controller nlpsolve (ipopt, nlpsol_sfun, v2)"/2
  [en_arr] -> Selector2/1
  Selector2/1 -> "MPC1 offline controller nlpsolve (ipopt, nlpsol_sfun, v2)"/Enable
  "MPC1 offline controller nlpsolve (ipopt, nlpsol_sfun, v2)"/1 -> [tau_MPC1]
  "MPC1 offline controller nlpsolve (ipopt, nlpsol_sfun, v2)"/2 -> [x_d_trj_MPC1]
  idx3/1 -> Selector2/2
  "MPC1 offline controller nlpsolve (ipopt, nlpsol_sfun, v2)"/3 -> [debug_data_MPC1]
  [robot_model] -> "MPC1 offline controller nlpsolve (ipopt, nlpsol_sfun, v2)"/1
  idx2/1 -> Selector5/2
  [robot_model] -> "MPC2 offline controller nlpsolve (qrqp, nlpsol_sfun, v2)"/1
  [en_arr] -> Selector5/1
  Selector5/1 -> "MPC2 offline controller nlpsolve (qrqp, nlpsol_sfun, v2)"/Enable
  "MPC2 offline controller nlpsolve (qrqp, nlpsol_sfun, v2)"/2 -> [x_d_trj_MPC2]
  "MPC2 offline controller nlpsolve (qrqp, nlpsol_sfun, v2)"/1 -> [tau_MPC2]
  [traj_select] -> "MPC2 offline controller nlpsolve (qrqp, nlpsol_sfun, v2)"/2
  "MPC2 offline controller nlpsolve (qrqp, nlpsol_sfun, v2)"/3 -> [debug_data_MPC2]
  [robot_model] -> "MPC3 offline controller nlpsolve (qrqp, nlpsol_sfun, v3)"/1
  [en_arr] -> Selector3/1
  "MPC3 offline controller nlpsolve (qrqp, nlpsol_sfun, v3)"/2 -> [x_d_trj_MPC3]
  [traj_select] -> "MPC3 offline controller nlpsolve (qrqp, nlpsol_sfun, v3)"/2
  "MPC3 offline controller nlpsolve (qrqp, nlpsol_sfun, v3)"/3 -> [debug_data_MPC3]
  "MPC3 offline controller nlpsolve (qrqp, nlpsol_sfun, v3)"/1 -> [tau_MPC3]
  Selector3/1 -> "MPC3 offline controller nlpsolve (qrqp, nlpsol_sfun, v3)"/Enable
  idx1/1 -> Selector3/2
  [en_arr] -> Selector4/1
  "MPC4 offline controller nlpsolve (qrqp, opti_sfun, v1)"/2 -> [x_d_trj_MPC4]
  Selector4/1 -> "MPC4 offline controller nlpsolve (qrqp, opti_sfun, v1)"/Enable
  "MPC4 offline controller nlpsolve (qrqp, opti_sfun, v1)"/1 -> [tau_MPC4]
  "MPC4 offline controller nlpsolve (qrqp, opti_sfun, v1)"/3 -> [debug_data_MPC4]
  idx4/1 -> Selector4/2
  [robot_model] -> "MPC4 offline controller nlpsolve (qrqp, opti_sfun, v1)"/1
  [traj_select] -> "MPC4 offline controller nlpsolve (qrqp, opti_sfun, v1)"/2
  idx5/1 -> Selector6/2
  "MPC5 offline controller nlpsolve (qrqp, nlpsol_sfun)"/1 -> [tau_MPC5]
  Selector6/1 -> "MPC5 offline controller nlpsolve (qrqp, nlpsol_sfun)"/Enable
  "MPC5 offline controller nlpsolve (qrqp, nlpsol_sfun)"/3 -> [debug_data_MPC5]
  [traj_select] -> "MPC5 offline controller nlpsolve (qrqp, nlpsol_sfun)"/2
  "MPC5 offline controller nlpsolve (qrqp, nlpsol_sfun)"/2 -> [x_d_trj_MPC5]
  [en_arr] -> Selector6/1
  [robot_model] -> "MPC5 offline controller nlpsolve (qrqp, nlpsol_sfun)"/1
  [debug_data_MPC5] -> Merge/6
  [x_d_trj_MPC5] -> Merge2/6
  [tau_MPC5] -> Merge1/6

== system sim_discrete_planar_7dof/tic-toc/tic-toc ==
  Trigger : TriggerPort  VariantControl=(inherit)
  MATLAB Function : MATLAB Function  TreatAsAtomicUnit=on

== system sim_discrete_planar_7dof/Debug Subsystem/messages on end/output debug text ==
  x_err_mean : Inport
  y_err_mean : Inport  Port=2
  Trigger : TriggerPort  VariantControl=(inherit)
  MATLAB Function : MATLAB Function  TreatAsAtomicUnit=on
  wires:
  y_err_mean/1 -> MATLAB Function/2(y_err_mean)
  x_err_mean/1 -> MATLAB Function/1(x_err_mean)

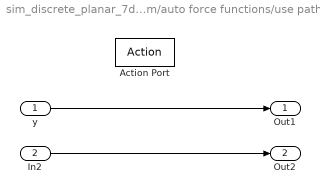
== system sim_discrete_planar_7dof/External force subsystem/auto force functions/use path poly ==
  y : Inport
  In2 : Inport  Port=2
  Action Port : ActionPort
  Out1 : Outport
  Out2 : Outport  Port=2
  wires:
  In2/1 -> Out2/1
  y/1 -> Out1/1

== system sim_discrete_planar_7dof/External force subsystem/auto force functions/use welder path ori ==
  custom_mode : Inport
  In2 : Inport  Port=2
  Action Port : ActionPort
  Out1 : Outport
  Out2 : Outport  Port=2
  wires:
  custom_mode/1 -> Out1/1
  In2/1 -> Out2/1

== system sim_discrete_planar_7dof/External force subsystem/auto force functions/use welder path snap ==
  custom_mode : Inport
  In2 : Inport  Port=2
  Action Port : ActionPort
  Out1 : Outport
  Out2 : Outport  Port=2
  wires:
  In2/1 -> Out2/1
  custom_mode/1 -> Out1/1

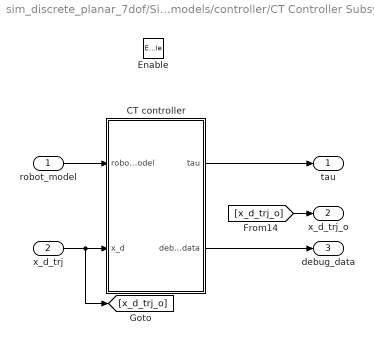
== system sim_discrete_planar_7dof/Simulation models/controller/CT Controller Subsystem ==
  robot_model : Inport  OutDataTypeStr=Bus: robot_model
  x_d_trj : Inport  Port=2  OutDataTypeStr=Bus: x_d
  Enable : EnablePort
  CT controller : MATLAB Function  TreatAsAtomicUnit=on
  tau : Outport
  x_d_trj_o : Outport  Port=2  OutDataTypeStr=Bus: x_d
  debug_data : Outport  Port=3  OutDataTypeStr=Bus: debug_data_bus
  wires:
  robot_model/1 -> CT controller/1(robot_model)
  x_d_trj/1 -> CT controller/2(x_d), [x_d_trj_o]
  CT controller/1(tau) -> tau/1
  CT controller/2(debug_data) -> debug_data/1
  [x_d_trj_o] -> x_d_trj_o/1

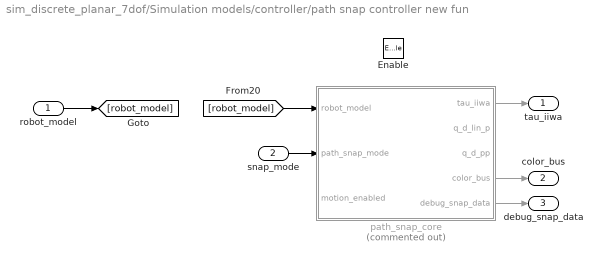
== system sim_discrete_planar_7dof/Simulation models/controller/path snap controller new fun ==
  robot_model : Inport
  snap_mode : Inport  Port=2
  Enable : EnablePort
  path_snap_core : MATLAB Function  Commented=on  TreatAsAtomicUnit=on
  tau_iiwa : Outport
  color_bus : Outport  Port=2  OutDataTypeStr=Bus: color_bus
  debug_snap_data : Outport  Port=3  OutDataTypeStr=Bus: debug_snap_data_bus
  wires:
  path_snap_core/4(color_bus) -> color_bus/1
  path_snap_core/1(tau_iiwa) -> tau_iiwa/1
  snap_mode/1 -> path_snap_core/2(path_snap_mode)
  [robot_model] -> path_snap_core/1(robot_model)
  robot_model/1 -> [robot_model]
  path_snap_core/5(debug_snap_data) -> debug_snap_data/1

== matlab function sim_discrete_planar_7dof/Simulation models/Robot model/Reduziertes System ==
  data: tau input; q_pp output; q input; q_p input; param_robot parameter
function q_pp =fcn(tau, q, q_p, param_robot)

M=inertia_matrix(q,param_robot);                          % rigid body inertia matrix
C=coriolis_matrix(q,q_p,param_robot);                     % coriolis matrix
g=gravitational_forces(q,param_robot);                    % gravitational forces

q_pp = M\(tau - C*q_p - g);

% q_pp = M\(tau-C*q_p-g - 0.5*diag(ones(7,1))*q_p(3:9)); % mit Reibung

== matlab function sim_discrete_planar_7dof/External force subsystem/external_force ==
  settings: updateMethod=DISCRETE  sampleTime=param_global.Ta
  data: f_W_E input; robot_model input; debug_snap_data input Bus: debug_snap_data_bus; tau_ext output; mode input; f_ext output
function [tau_ext, f_ext] = fcn(f_W_E, robot_model, debug_snap_data, mode)
    if(mode == 1) % Kraft ist im Weltsystem definiert
        f_ext = f_W_E; %Externe Kraft / Moment in Welt KOS definiert
    elseif(mode == 2) % Externe Kraft / Moment in Endeffektor KOS definiert
        % Rechnet die Kräfte im Weltsystem die auf den Endeffektor um in Kräfte,
        % die im Endeffektorsystem direkt auf den Endeffektor wirken, damit eine
        % intuitiverer Steuerung möglich ist (Der Benutzer legt ja auch die Kräfte
        % aus Sicht des Endeffektorsystem an und nicht aus Sicht des Weltsystems)
        
        R_W_E = robot_model.H(1:3,1:3);
        
        % indizes nicht ganz logisch
        F_W_E = f_W_E(1:3);
        tau_W_E = f_W_E(4:6);
        
        
        F_E_E = R_W_E*F_W_E;
        tau_E_E = R_W_E*tau_W_E;
        
        f_ext = [F_E_E;tau_E_E];
    else % Externe Kraft im Pfadkoordinatensystem des aktiven Pfads
        F_W_E = f_W_E(1:3);
        tau_W_E = f_W_E(4:6);
        active_path_index_t = debug_snap_data.active_path_index_t;
        if(active_path_index_t == 0) % if CT CONTROL TODO: Problem bei orienation snap wenn path index > N_path ist.
            R_W_path = eye(3);
        else
            R_W_path = debug_snap_data.Rot_transport_frame(:,:,active_path_index_t); % only active path
        end

        F_path_E = R_W_path*F_W_E;
        tau_path_E = R_W_path*tau_W_E;
        
        f_ext = [F_path_E;tau_path_E];
    end
    %theta_star = debug_snap_data.theta_star;
    %N_path = param_global.N_path;

    %R_W_path = debug_snap_data.Rot_transport_frame; % all paths
    %path_frame_position = zeros(3,2,N_path);
    %for i=1:1:N_path
    %    [sigma, ~, ~, ~] = eval_path_t(theta_star(i), i, path_param);
    %    path_frame_position(:,:,i) = [sigma rotm2eul(R_W_path(:,:,i), 'XYZ')];
    %end

    J = robot_model.J;
    tau_ext_temp = J' * f_ext;
    tau_ext = tau_ext_temp(3:9);
end

== matlab function sim_discrete_planar_7dof/Simulation models/controller/Controller Enable ==
  settings: sampleTime=param_global.Ta
  data: en_arr output; selector input uint32
function en_arr  = fcn(selector)
    % Wichtig: selector \in [1,max(selector)]
    % Es wird ein bool array ausgegeben, welches nur den index 1 setzt, der
    % mit selector übereinstimmt. Achtung: Size von "en_arr" muss
    % entsprechend der Ausgänge unter "Edit Data" manuell angegeben werden.
    % Beispiel: 4 Inputs, max(selector)=4, Size = [1 4]
    % z. B. selector = 2
    % 1:4 == selector liefert [0 1 0 0]
    en_arr = (1:6 == selector)';
end

== matlab function sim_discrete_planar_7dof/External force subsystem/auto force functions/get signals ==
  data: t input; y output size=6; t0 input; y0 input; m0 input; custom_mode output
function [y,custom_mode] = fcn(t, t0, y0, m0)
% ti_a ... Anfangszeit
% ti_e ... Endzeit
% yi ... Pulswert
% mi ... mode: 1 if f_w_e, 2 if f_e_e, 3 if f_path
% outputs
% y ... chosen Pulswert
% custom mode: chose mode

i = sum(t >= t0);
y = y0(i,:)';
custom_mode = m0(i);

== matlab function sim_discrete_planar_7dof/External force subsystem/auto force functions/get signals1 ==
  data: t input; y output size=6; t0_a input; t0_e input; y0 input; m0 input; t1_a input; t1_e input; y1 input; m1 input; t2_a input; t2_e input; y2 input; m2 input; t3_a input; t3_e input; y3 input; m3 input; t4_a input; t4_e input; y4 input; custom_mode output; m4 input
function [y,custom_mode] = fcn(t, t0_a, t0_e, y0, m0, t1_a, t1_e, y1, m1, t2_a, t2_e, y2, m2, t3_a, t3_e, y3, m3, t4_a, t4_e, y4, m4)
% ti_a ... Anfangszeit
% ti_e ... Endzeit
% yi ... Pulswert
% mi ... mode: 1 if f_w_e, 2 if f_e_e, 3 if f_path
% outputs
% y ... chosen Pulswert
% custom mode: chose mode

if(t >= t0_a && t < t0_e)
    y = y0;
    custom_mode = m0; % f_path
elseif(t >= t1_a && t < t1_e)
    y = y1;
    custom_mode = m1; % f_e_e
elseif(t >= t2_a && t < t2_e)
    y = y2;
    custom_mode = m2; % f_path
elseif(t >= t3_a && t < t3_e)
    y = y3;
    custom_mode = m3; % f_path
elseif(t >= t4_a && t < t4_e)
    y = y4;
    custom_mode = m4; % f_path
else
    y = [0 0 0 0 0 0]';
    custom_mode = 1; % f_w_e
end

== matlab function sim_discrete_planar_7dof/External force subsystem/auto force functions/get signals2 ==
  data: t input; y output size=6; t0 input; y0 input; m0 input; custom_mode output
function [y,custom_mode] = fcn(t, t0, y0, m0)
% ti_a ... Anfangszeit
% ti_e ... Endzeit
% yi ... Pulswert
% mi ... mode: 1 if f_w_e, 2 if f_e_e, 3 if f_path
% outputs
% y ... chosen Pulswert
% custom mode: chose mode

i = sum(t >= t0);
y = y0(i,:)';
custom_mode = m0(i);

== matlab function sim_discrete_planar_7dof/Simulation models/Robot model bus ==
  settings: updateMethod=DISCRETE  sampleTime=param_global.Ta
  data: q input; q_p input; q_pp input; robot_model output Bus: robot_model; param_robot parameter
function robot_model = fcn(q, q_p, q_pp, param_robot)
% Parameters
robot_model=struct();
robot_model.q=q;                    % generalized coordinates
robot_model.q_p=q_p;                % time derivative of generalized coordinates
robot_model.q_pp=q_pp;
robot_model.H=hom_transform_endeffector(q, param_robot);            % homogenous transformation to end-effector
robot_model.J=geo_jacobian_endeffector(q,param_robot);              % geometric jacobian to end-effector
robot_model.J_p=geo_jacobian_endeffector_p(q, q_p,param_robot);     % time derivative of geometric jacobian to end-effector
robot_model.M=inertia_matrix(q,param_robot);                        % inertia matrix
robot_model.C=coriolis_matrix(q, q_p,param_robot);                  % coriolis matrix
robot_model.g=gravitational_forces(q,param_robot);                  % gravitational forces
end

== matlab function sim_discrete_planar_7dof/tic-toc/MATLAB Function ==
  settings: updateMethod=DISCRETE  sampleTime=param_global.Ta
  data: t input; param_vis parameter
function fcn(t, param_vis)

if(t==0)
    tic;
end

if(t==param_vis.T)
    toc;
end

== matlab function sim_discrete_planar_7dof/Debug Subsystem/messages on end/MATLAB Function ==
  settings: updateMethod=DISCRETE  sampleTime=param_global.Ta
  data: t input; param_vis parameter
function fcn(t, param_vis)

if(t==0)
    tic;
end

if(t==param_vis.T)
    toc;
end

== matlab function sim_discrete_planar_7dof/tic-toc/tic-toc/MATLAB Function ==
  settings: updateMethod=DISCRETE
function fcn()
persistent flag;

if(isempty(flag))
    flag=0;
end

if(flag == 0)
    tic
    flag=1;
else
    disp(['Simulink execution time: ', sprintf('%f', toc), ' s']);
end

== matlab function sim_discrete_planar_7dof/Debug Subsystem/messages on end/output debug text/MATLAB Function ==
  settings: updateMethod=DISCRETE
  data: x_err_mean input; y_err_mean input
function fcn(x_err_mean, y_err_mean)
    disp(['mean x_err = ', sprintf('%g', x_err_mean), ' m']);
    disp(['mean y_err = ', sprintf('%g', y_err_mean), ' m']);
end

== matlab function sim_discrete_planar_7dof/Debug Subsystem/MATLAB Function ==
  data: x_err_mean_out output; x_err input; y_err input; y_err_mean_out output
function [x_err_mean_out, y_err_mean_out] = fcn(x_err, y_err)

persistent cnt;
persistent x_err_mean;
persistent y_err_mean;

if(isempty(cnt))
    cnt = 1;
    x_err_mean = 0;
    y_err_mean = 0;
end
% m1 =  a          = (0*m0+a)/1
% m2 = (a+b)/2     = (1*m1+b)/2
% m3 = (a+b+c)/3   = (2*m2+c)/3
% m4 = (a+b+c+d)/4 = (3*m3+d)/4
% ...
% mi = ((i-1)*m_{i-1})/i; 
x_err_mean = ((cnt-1)*x_err_mean + x_err)/cnt;
y_err_mean = ((cnt-1)*y_err_mean + y_err)/cnt;

x_err_mean_out = x_err_mean;
y_err_mean_out = y_err_mean;

cnt = cnt + 1;

%Die iterative Methode ist anfälliger für Rundungsfehler.
%Die iterative Methode kann bei sehr großen Datenmengen numerisch instabil
% werden

== matlab function sim_discrete_planar_7dof/Simulation models/controller/CT Controller Subsystem/CT controller ==
  settings: updateMethod=DISCRETE  sampleTime=param_global.Ta
  data: tau output; robot_model input Bus: robot_model; x_d input Bus: x_d; ct_ctrl_param parameter; debug_data output Bus: debug_data_bus
function [tau, debug_data] = fcn(robot_model, x_d, ct_ctrl_param)

% Parameters
%q = robot_model.q;      % generalized coordinates
q_p = robot_model.q_p;  % time derivative of generalized coordinates
q_pp = robot_model.q_pp;
M = robot_model.M;      % inertia matrix
C = robot_model.C;      % coriolis matrix
g = robot_model.g;      % gravitational forces
J = robot_model.J;      % geometric jacobian to end-effector
J_p = robot_model.J_p;  % time derivative of geometric jacobian to end-effector
H = robot_model.H;

J_v   = J(1:2, 1:2);
J_v_p = J_p(1:2, 1:2);

% Current Trajectory
p    = H(1:2,4);
p_p  = J_v*q_p;
p_pp = J_v*q_pp + J_v_p*q_p;

% Desired Trajectory
p_d    = x_d.p_d(1:2);
p_d_p  = x_d.p_d_p(1:2);
p_d_pp = x_d.p_d_pp(1:2);

% Control parameters
% kartesisch
Kp1 = ct_ctrl_param.Kp1;
Kd1 = ct_ctrl_param.Kd1;

% CT control law
%% Cartesian Endeffector Pose
%x_err = [ p- x_d.p_d; q_err(2:4)'];   % Error as quaternion
%x_err_p = [p_p - x_d.p_d_p; omega_e - x_d.omega_d];
%v = J\(x_d_pp  - Kd1*x_err_p - Kp1*x_err - J_p*q_p);
%v = inv(J(1:2,1:2))*(x_d_pp(1:2)  - Kd1(1:2,1:2)*x_err_p(1:2) - Kp1(1:2,1:2)*x_err(1:2) - J_p(1:2,1:2)*q_p);
sing_method = ct_ctrl_param.mode;

if(sing_method == 0)
    v = J_v\(p_d_pp - Kd1*(p_p - p_d_p) - Kp1*(p - p_d) - J_v_p*q_p);
elseif(sing_method == 1) % add +k*E
    k = ct_ctrl_param.k;
    J_pinv = (J_v'*J_v + k*eye(2))\J_v';
    v = J_pinv*(p_d_pp - Kd1*(p_p - p_d_p) - Kp1*(p - p_d) - J_v_p*q_p);
elseif(sing_method == 2) % add +lambda*E
    w_bar_N = ct_ctrl_param.w_bar_N;
    w_E = ct_ctrl_param.w_E;

    W_E = w_E.*diag([1 1]);
    e = (p - p_d);
    E_k = 1/2*e' * W_E * e;
    W_N = diag(E_k + w_bar_N);

    [U, S, V] = svd(sqrt(W_E)*J_v);

    %H_k = V*(S^2 + W_N)*V'; % geht nur wenn alle w_n gleich sind
    H_k = V*(S^2)*V' + W_N;
    J_pinv = H_k\J_v';
    v = J_pinv*(p_d_pp - Kd1*(p_p - p_d_p) - Kp1*(p - p_d) - J_v_p*q_p);

    %J_pinv = (J_v'*W_E*J_v + W_N)\J_v';
    %v = J_pinv*(p_d_pp - Kd1*(p_p - p_d_p) - Kp1*(p - p_d) - J_v_p*q_p);
    
    %J_new = (J_v'*W_E*J_v + W_N);
    %v = J_new\(p_d_pp - Kd1*(p_p - p_d_p) - Kp1*(p - p_d) - J_v_p*q_p);
else % remove small singular values
    % Perform SVD
    [U, S, V] = svd(J_v);
    
    % Set a threshold for small singular values
    epsilon = ct_ctrl_param.eps; % Adjust epsilon as needed
    
    % Threshold small singular values in S
    S_new = diag(max(diag(S), epsilon));  % Creates a diagonal matrix with thresholded values
    
    % Reconstruct the matrix with modified singular values
    J_new = U * S_new * V';
    v = J_new\(p_d_pp - Kd1*(p_p - p_d_p) - Kp1*(p - p_d) - J_v_p*q_p);
end

tau = M*v + C*q_p + g;

%% DEBUG
debug_data.p    = p;
debug_data.p_p  = p_p;
debug_data.p_pp = p_pp;
debug_data.rot_x_err = 0;
debug_data.rot_y_err = 0;
debug_data.rot_z_err = 0;

== matlab function sim_discrete_planar_7dof/Debug Subsystem/comp vel and acc ==
  settings: updateMethod=CONTINUOUS  sampleTime=inf
  data: robot_model input Bus: robot_model; p output; param_robot parameter; x_d_trj input Bus: x_d; tau input; p_d output; p_p output; p_d_p output; p_pp output; p_d_pp output
function [p, p_d, p_p, p_d_p, p_pp, p_d_pp]  = fcn(robot_model, param_robot, x_d_trj, tau)

q = robot_model.q;
q_p = robot_model.q_p;

%%
M=inertia_matrix(q,param_robot);                          % rigid body inertia matrix
C=coriolis_matrix(q,q_p,param_robot);                     % coriolis matrix
g=gravitational_forces(q,param_robot);                    % gravitational forces

% Equations of motion
%tau_lin = [Mrr,Mrq]*q_d_pp + [Crr,Crq]*q_p + g(1:2);
%q_pp = M\([tau_lin;tau_iiwa]-C*q_p-g);

q_pp = M\(tau -C*q_p - g);

%%

%q_pp = robot_model.q_pp;

H = hom_transform_endeffector(q, param_robot);
J = robot_model.J;
J_p = robot_model.J_p;

p = H(1:2, 4);
p_p = J(1:2,:)*q_p;
p_pp = J(1:2,:)*q_pp + J_p(1:2,:)*q_p;

p_d = x_d_trj.p_d(1:2);
p_d_p = x_d_trj.p_d_p(1:2);
p_d_pp = x_d_trj.p_d_pp(1:2);

== matlab function sim_discrete_planar_7dof/Debug Subsystem/manipulability ==
  settings: sampleTime=param_global.Ta
  data: robot_model input; w output
function w  = manipulability(robot_model)

J = robot_model.J(1:2,1:2);
det_J = det(J*J');
w = sqrt(abs(det_J));
%q = robot_model.q;
%qnorm = sum(q.^2);

== matlab function sim_discrete_planar_7dof/Debug Subsystem/get pos ==
  settings: updateMethod=DISCRETE  sampleTime=param_global.Ta
  data: q input; yy_debug output Bus: yy_debug_bus; param_robot parameter; x_d_trj input Bus: x_d; init_bus_param parameter
function yy_debug  = fcn(q, param_robot, x_d_trj, init_bus_param)

yy_debug = init_bus_param.init_yy_debug_bus;

H = hom_transform_endeffector(q, param_robot);
y_t_W_E = H(1:3,4);
y_t_W_E_d = x_d_trj.p_d;

R_W_E = H(1:3,1:3);
ori_t_W_E = rotm2eul(R_W_E, 'XYZ');
ori_t_W_E_d = rotm2eul(quaternion2rotation(x_d_trj.q_d), 'XYZ');

yy_debug.x =  y_t_W_E(1);
yy_debug.x_d = y_t_W_E_d(1);

yy_debug.y =  y_t_W_E(2);
yy_debug.y_d = y_t_W_E_d(2);

yy_debug.z =  y_t_W_E(3);
yy_debug.z_d = y_t_W_E_d(3);

yy_debug.phi = ori_t_W_E(1);
yy_debug.phi_d = ori_t_W_E_d(1);

yy_debug.theta = ori_t_W_E(2);
yy_debug.theta_d = ori_t_W_E_d(2);

yy_debug.psi = ori_t_W_E(3);
yy_debug.psi_d = ori_t_W_E_d(3);

quat_err = quat_mult(rotation2quaternion(R_W_E), quat_inv(x_d_trj.q_d));
yy_debug.rot_x_err = quat_err(2);
yy_debug.rot_y_err = quat_err(3);
yy_debug.rot_z_err = quat_err(4);
